simulink model "WDGBrakingController"  (R2024a)
settings: configuration reference "csMultiInstance" (kept outside this file)
Description:
  | WDG Braking Controller (SW Component)
settings Model: DataDictionary=DD_WDGBrakingController.sldd  EnableAccessToBaseWorkspace=off  Creator=The MathWorks, Inc.  LastModifiedBy=The MathWorks, Inc.
settings ConfigSetRef: SourceName=csMultiInstance

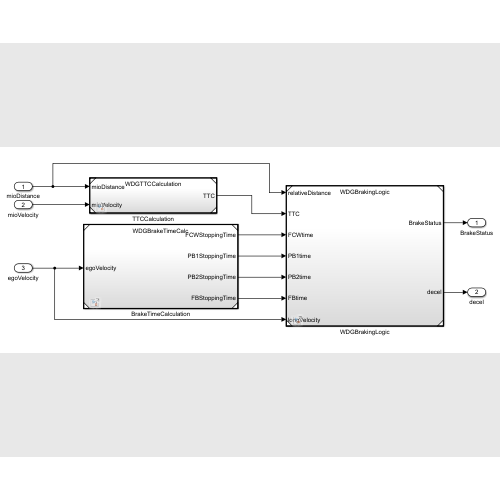
[thumbnail: Simulink's stored preview of the top-level diagram]
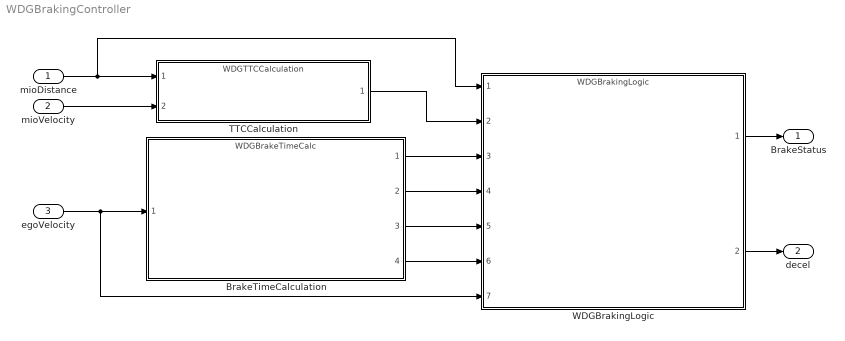
== system WDGBrakingController ==
  mioDistance : Inport
  mioVelocity : Inport  Port=2
  egoVelocity : Inport  Port=3
  BrakeTimeCalculation : ModelReference  ModelNameDialog=WDGBrakeTimeCalc  SimulationMode=Normal  ModelReferenceVersion=8.0
  TTCCalculation : ModelReference  ModelNameDialog=WDGTTCCalculation  SimulationMode=Normal  ModelReferenceVersion=8.0
  WDGBrakingLogic : ModelReference  ModelNameDialog=WDGBrakingLogic  SimulationMode=Normal  ModelReferenceVersion=8.0
  BrakeStatus : Outport
  decel : Outport  Port=2
  wires:
  TTCCalculation/1 -> WDGBrakingLogic/2
  BrakeTimeCalculation/1 -> WDGBrakingLogic/3
  BrakeTimeCalculation/2 -> WDGBrakingLogic/4
  BrakeTimeCalculation/3 -> WDGBrakingLogic/5
  BrakeTimeCalculation/4 -> WDGBrakingLogic/6
  mioDistance/1 -> WDGBrakingLogic/1, TTCCalculation/1
  mioVelocity/1 -> TTCCalculation/2
  egoVelocity/1 -> WDGBrakingLogic/7, BrakeTimeCalculation/1
  WDGBrakingLogic/1 -> BrakeStatus/1
  WDGBrakingLogic/2 -> decel/1
